simulink model "observer"  (R2022b)
settings: Solver=VariableStepAuto  StartTime=0.0  StopTime=5000  RelTol=1e-3
libraries: mssSimulink x2
settings Model: Creator=ADMIN  LastModifiedBy=ADMIN

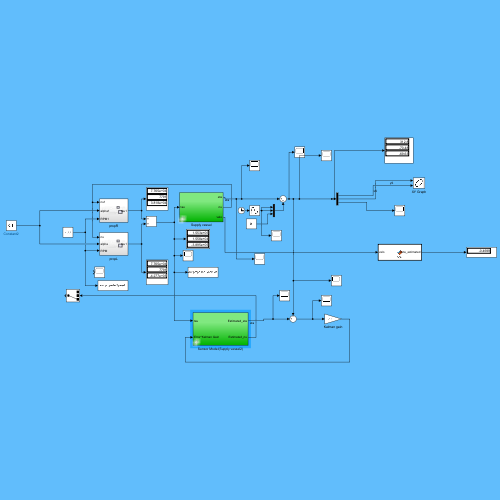
[thumbnail: Simulink's stored preview of the top-level diagram]
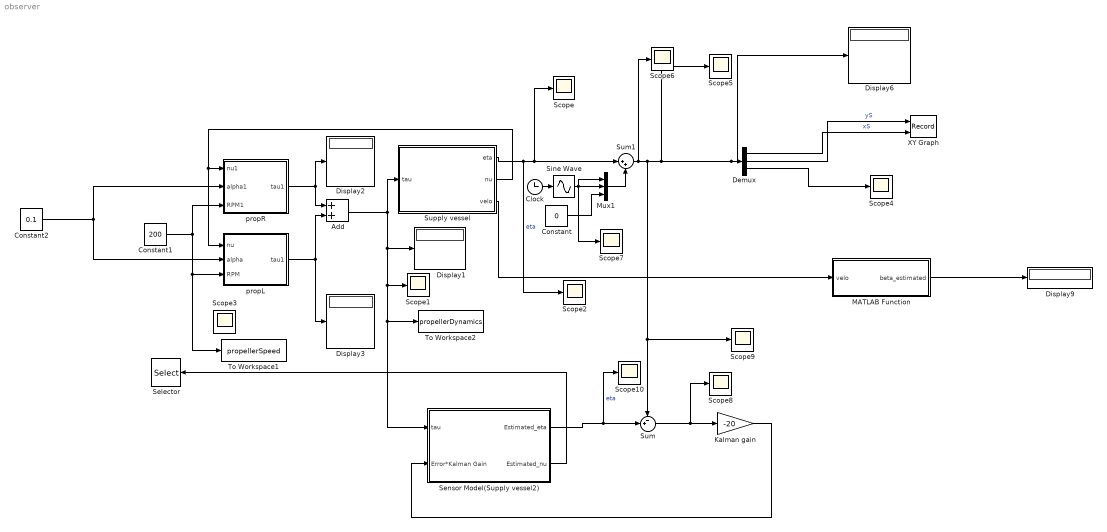
== system observer ==
  Add : Sum
  Clock : Clock
  Constant : Constant  Value=0
  Constant1 : Constant  Value=200
  Constant2 : Constant  Value=0.1
  Demux : Demux  Outputs=3
  Display{1..3,6,9} (5 alike) : Display
  Kalman gain : Gain  Gain=-20
  MATLAB Function : MATLAB Function  TreatAsAtomicUnit=on
  Mux1 : Mux  Inputs=3
  Scope{,1..10} (11 alike) : Scope
  Selector : Selector  InputPortWidth=3  IndexOptions=Index vector (dialog)  Indices=[3]  OutputSizes=1
  Sensor Model(Supply vessel2) : Subsystem  AncestorBlock=mssSimulink/Marine craft models/Supply vessel
      settings: LibrarySourceBlock=mssSimulink/Marine craft models/Supply vessel
  Sine Wave : Sin  TimeSource=Use external signal  SampleTime=0
  Sum : Sum  Inputs=-+|
  Sum1 : Sum  Inputs=|++
  Supply vessel : Subsystem  AncestorBlock=mssSimulink/Marine craft models/Supply vessel
      settings: LibrarySourceBlock=mssSimulink/Marine craft models/Supply vessel
  To Workspace1 : ToWorkspace  VariableName=propellerSpeed  SaveFormat=Timeseries  SampleTime=-1
  To Workspace2 : ToWorkspace  VariableName=propellerDynamics  SaveFormat=Timeseries  SampleTime=-1
  XY Graph : Record  FileSettingsInternal="{\"entries\":[{\"content\":{\"excelSettings\":{\"content\":{},\"type\":\"Streamout.ExcelSettings\"}},\"type\":\"Streamout.FileSettingStorage\",\"uuid\":\"745f10b0-d431-460f-8bac-5fec13218052\"}],\"packageUris\":[\"http://schema.mathworks.com/mf0/streamout_blocks/R2020a\"],\"version\":\"1.0\"}"  Layout=[1 1]  SignalsInternal="{\"entries\":[{\"content\":{\"signals\":[{\"content\":{\"blockPath\":[\"untitled/XY Graph\"],\"channel\":[],\"dimensions\":[1],\"domain\":\"untitled/XY Graph\",\"lineColor\":\"#edb120\",\"plots\":[],\"port\":1,\"sid\":[\"\"],\"signalID\":6053,\"signalName\":\"yS\"},\"type\":\"RecordBlkView.Signal\",\"uuid\":\"76aacf64-0f69-4baf-8ee2-86f53dc3926d\"},{\"content\":{\"blockPath\":[\"untitled/XY Graph\"],\"channel\":[],\"dimensions\":[1],\"domain\":\"untitled/XY Graph\",\"lineColor\":\"#7e2f8e\",\"plots\":[],\"port\":2,\"sid\":[\"\"],\"signalID\":6057,\"signalName\":\"xS\"},\"type\":\"RecordBlkView.Signal\",\"uuid\":\"9f0f96a2-05ba-4d7f-9a6e-25fee0664970\"}]},\"type\":\"RecordBlkView.InputSignals\",\"uuid\":\"3a7a1a35-8a4d-4271-a4b4-a2beea98fdd3\"}],\"packageUris\":[\"http://schema.mathworks.com/mf0/streamout_blocks/R2020a\"],\"version\":\"1.0\"}"  VisualizationBindings="{\"xyplotplugin\":{\"info\":[{\"series\":[],\"subplotID\":1}]}}"  CompatibilityTag=XY
  propL : Subsystem
  propR : Subsystem
  wires:
  Sum1/1 -> Scope6/1, Scope5/1, Demux/1, Display6/1, Sum/1, Scope9/1
  Sine Wave/1 -> Scope7/1, Mux1/2, Mux1/1
  Mux1/1 -> Sum1/2
  propL/1(tau1) -> Add/2, Display3/1
  Sensor Model(Supply vessel2)/2(Estimated_nu) -> Selector/1
  Demux/1 -> XY Graph/2  "xS"
  Sum/1 -> Scope8/1, Kalman gain/1
  Sensor Model(Supply vessel2)/1(Estimated_eta) -> Scope10/1, Sum/2  "eta"
  Supply vessel/1(eta) -> Sum1/1, Scope/1, Scope2/1  "eta"
  Kalman gain/1 -> Sensor Model(Supply vessel2)/2(Error*Kalman Gain)
  Supply vessel/3(velo) -> MATLAB Function/1(velo)
  Demux/3 -> Scope4/1
  Demux/2 -> XY Graph/1  "yS"
  Supply vessel/2(nu) -> propR/1(nu1), propL/1(nu)
  Clock/1 -> Sine Wave/1
  propR/1(tau1) -> Display2/1, Add/1
  Add/1 -> Sensor Model(Supply vessel2)/1(tau), To Workspace2/1, Scope1/1, Display1/1, Supply vessel/1(tau)
  MATLAB Function/1(beta_estimated) -> Display9/1
  Constant/1 -> Mux1/3
  Constant1/1 -> propL/3(RPM), To Workspace1/1, propR/3(RPM1)
  Constant2/1 -> propL/2(alpha), propR/2(alpha1)

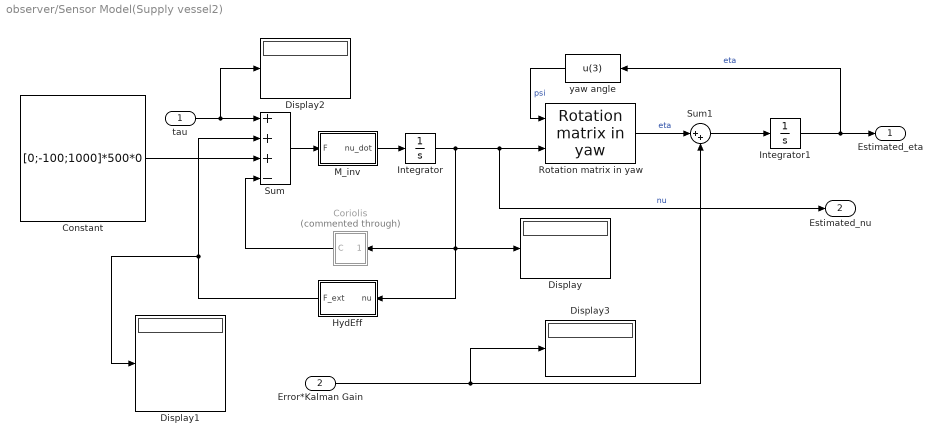
== system observer/Sensor Model(Supply vessel2) ==
  tau : Inport
  Error*Kalman Gain : Inport  Port=2
  Constant : Constant  Value=[0;-100;1000]*500*0
  Coriolis : Subsystem  Commented=through
  Display{,1..3} (4 alike) : Display
  HydEff : Subsystem
  Integrator : Integrator  InitialCondition=[0 1 0]
  Integrator1 : Integrator
  M_inv : Subsystem
  "Rotation matrix in yaw " : mssSimulink/Modelling/Kinematics/Rotation matrix in yaw 
  Sum : Sum  Inputs=+++-  InputSameDT=on  SaturateOnIntegerOverflow=on  OutDataTypeStr=Inherit: Same as first input
  Sum1 : Sum  Inputs=|++
  yaw angle : Fcn  Expr=u(3)
  Estimated_eta : Outport  InitialOutput=0  VectorParamsAs1DForOutWhenUnconnected=off
  Estimated_nu : Outport  Port=2  InitialOutput=0  VectorParamsAs1DForOutWhenUnconnected=off
  wires:
  Sum/1 -> M_inv/1(F)
  M_inv/1(nu_dot) -> Integrator/1
  tau/1 -> Display2/1, Sum/1
  yaw angle/1 -> "Rotation matrix in yaw "/1  "psi"
  Integrator/1 -> Estimated_nu/1, "Rotation matrix in yaw "/2, Display/1, HydEff/1(nu), Coriolis/1(nu)  "nu"
  HydEff/1(F_ext) -> Display1/1, Sum/2
  Coriolis/1(C) -> Sum/4
  Constant/1 -> Sum/3
  Integrator1/1 -> Estimated_eta/1, yaw angle/1  "eta"
  Error*Kalman Gain/1 -> Display3/1, Sum1/2
  Sum1/1 -> Integrator1/1
  "Rotation matrix in yaw "/1 -> Sum1/1  "eta"

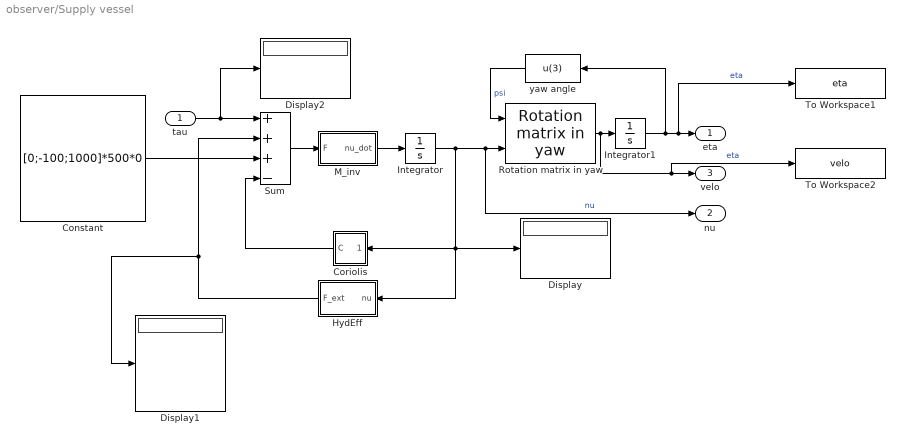
== system observer/Supply vessel ==
  tau : Inport
  Constant : Constant  Value=[0;-100;1000]*500*0
  Coriolis : Subsystem
  Display : Display
  Display1 : Display
  Display2 : Display
  HydEff : Subsystem
  Integrator : Integrator  InitialCondition=[0 1 0]
  Integrator1 : Integrator
  M_inv : Subsystem
  "Rotation matrix in yaw " : mssSimulink/Modelling/Kinematics/Rotation matrix in yaw 
  Sum : Sum  Inputs=+++-  InputSameDT=on  SaturateOnIntegerOverflow=on  OutDataTypeStr=Inherit: Same as first input
  To Workspace1 : ToWorkspace  VariableName=eta  SaveFormat=Timeseries  SampleTime=-1
  To Workspace2 : ToWorkspace  VariableName=velo  SaveFormat=Timeseries  SampleTime=-1
  yaw angle : Fcn  Expr=u(3)
  eta : Outport  InitialOutput=0  VectorParamsAs1DForOutWhenUnconnected=off
  nu : Outport  Port=2  InitialOutput=0  VectorParamsAs1DForOutWhenUnconnected=off
  velo : Outport  Port=3
  wires:
  Sum/1 -> M_inv/1(F)
  M_inv/1(nu_dot) -> Integrator/1
  tau/1 -> Display2/1, Sum/1
  yaw angle/1 -> "Rotation matrix in yaw "/1  "psi"
  Integrator/1 -> Display/1, HydEff/1(nu), Coriolis/1(nu), "Rotation matrix in yaw "/2, nu/1  "nu"
  HydEff/1(F_ext) -> Display1/1, Sum/2
  Coriolis/1(C) -> Sum/4
  Constant/1 -> Sum/3
  Integrator1/1 -> yaw angle/1, To Workspace1/1, eta/1  "eta"
  "Rotation matrix in yaw "/1 -> To Workspace2/1, velo/1, Integrator1/1  "eta"

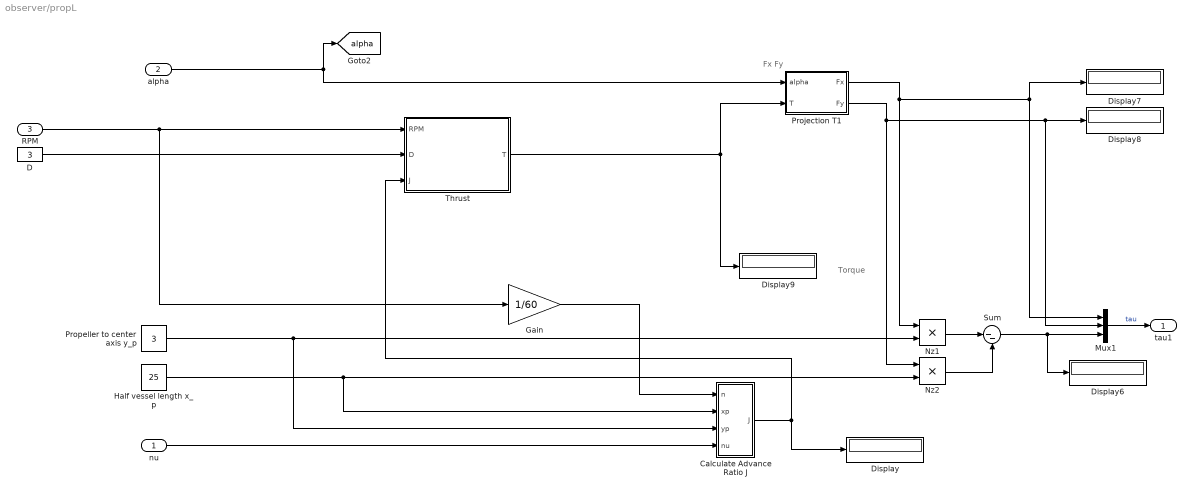
== system observer/propL ==
  note: Fx Fy
  note: Torque
  nu : Inport
  alpha : Inport  Port=2
  RPM : Inport  Port=3
  Calculate Advance Ratio J : Subsystem
  D : Constant  Value=3
  Display{,6..9} (5 alike) : Display
  Gain : Gain  Gain=1/60
  Half vessel length x_p : Constant  Value=25
  Mux1 : Mux  Inputs=3
  Nz1 : Product
  Nz2 : Product
  Projection T1 : MATLAB Function  TreatAsAtomicUnit=on
  Propeller to center axis y_p : Constant  Value=3
  Sum : Sum  Inputs=|--
  Thrust : Subsystem
  tau1 : Outport
  tag scope: alpha=global
  wires:
  Gain/1 -> Calculate Advance Ratio J/1(n)
  Thrust/1(T) -> Projection T1/2(T), Display9/1
  Propeller to center axis y_p/1 -> Calculate Advance Ratio J/3(yp), Nz1/2
  Projection T1/2(Fy) -> Mux1/2, Display8/1, Nz2/1
  RPM/1 -> Gain/1, Thrust/1(RPM)
  Nz2/1 -> Sum/2
  Projection T1/1(Fx) -> Display7/1, Mux1/1, Nz1/1
  Mux1/1 -> tau1/1  "tau"
  alpha/1 -> Projection T1/1(alpha), [alpha]
  D/1 -> Thrust/2(D)
  nu/1 -> Calculate Advance Ratio J/4(nu)
  Half vessel length x_p/1 -> Calculate Advance Ratio J/2(xp), Nz2/2
  Nz1/1 -> Sum/1
  Calculate Advance Ratio J/1(J) -> Thrust/3(J), Display/1
  Sum/1 -> Display6/1, Mux1/3

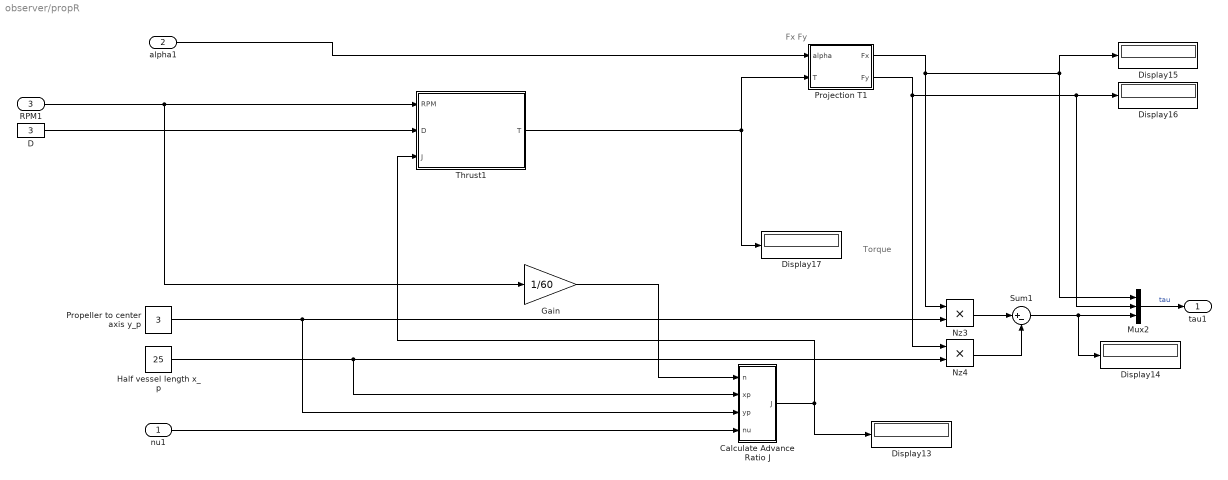
== system observer/propR ==
  note: Fx Fy
  note: Torque
  nu1 : Inport
  alpha1 : Inport  Port=2
  RPM1 : Inport  Port=3
  Calculate Advance Ratio J : Subsystem
  D : Constant  Value=3
  Display{13..17} (5 alike) : Display
  Gain : Gain  Gain=1/60
  Half vessel length x_p : Constant  Value=25
  Mux2 : Mux  Inputs=3
  Nz3 : Product
  Nz4 : Product
  Projection T1 : MATLAB Function  TreatAsAtomicUnit=on
  Propeller to center axis y_p : Constant  Value=3
  Sum1 : Sum  Inputs=|+-
  Thrust1 : Subsystem
  tau1 : Outport
  wires:
  Gain/1 -> Calculate Advance Ratio J/1(n)
  Thrust1/1(T) -> Projection T1/2(T), Display17/1
  Propeller to center axis y_p/1 -> Calculate Advance Ratio J/3(yp), Nz3/2
  Projection T1/2(Fy) -> Mux2/2, Display16/1, Nz4/1
  RPM1/1 -> Gain/1, Thrust1/1(RPM)
  Nz4/1 -> Sum1/2
  Projection T1/1(Fx) -> Display15/1, Mux2/1, Nz3/1
  Mux2/1 -> tau1/1  "tau"
  alpha1/1 -> Projection T1/1(alpha)
  D/1 -> Thrust1/2(D)
  nu1/1 -> Calculate Advance Ratio J/4(nu)
  Half vessel length x_p/1 -> Calculate Advance Ratio J/2(xp), Nz4/2
  Nz3/1 -> Sum1/1
  Calculate Advance Ratio J/1(J) -> Thrust1/3(J), Display13/1
  Sum1/1 -> Display14/1, Mux2/3

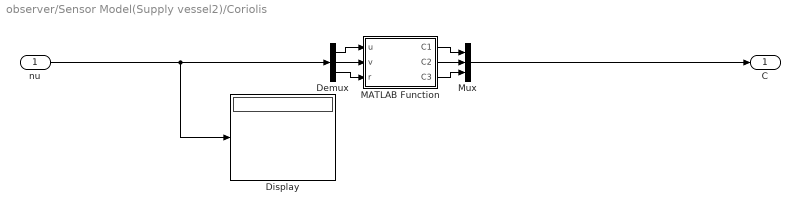
== system observer/Sensor Model(Supply vessel2)/Coriolis ==
  nu : Inport
  Demux : Demux  Outputs=3
  Display : Display
  MATLAB Function : MATLAB Function  TreatAsAtomicUnit=on
  Mux : Mux  Inputs=3
  C : Outport
  wires:
  nu/1 -> Display/1, Demux/1
  MATLAB Function/2(C2) -> Mux/2
  MATLAB Function/3(C3) -> Mux/3
  MATLAB Function/1(C1) -> Mux/1
  Mux/1 -> C/1
  Demux/1 -> MATLAB Function/1(u)
  Demux/2 -> MATLAB Function/2(v)
  Demux/3 -> MATLAB Function/3(r)

== system observer/Sensor Model(Supply vessel2)/HydEff ==
  nu : Inport
  Bus Creator : BusCreator  Inputs=3
  Demux : Demux  Outputs=3
  MATLAB Function : MATLAB Function  TreatAsAtomicUnit=on
  F_ext : Outport
  wires:
  [Mass1] -> MATLAB Function/1(mass)
  MATLAB Function/1(Xh) -> Bus Creator/1
  Bus Creator/1 -> F_ext/1
  MATLAB Function/2(Yh) -> Bus Creator/2
  MATLAB Function/3(Nh) -> Bus Creator/3
  nu/1 -> Demux/1
  Demux/1 -> MATLAB Function/2(u)
  Demux/2 -> MATLAB Function/3(v)
  Demux/3 -> MATLAB Function/4(r)

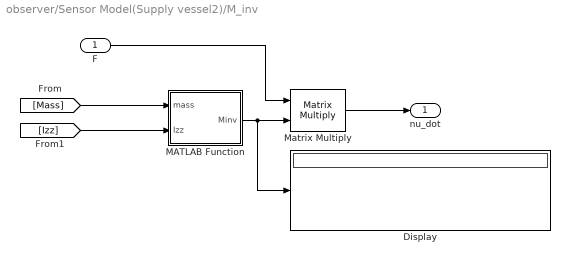
== system observer/Sensor Model(Supply vessel2)/M_inv ==
  F : Inport
  Display : Display
  MATLAB Function : MATLAB Function  TreatAsAtomicUnit=on
  Matrix Multiply : Product  Multiplication=Matrix(*)
  nu_dot : Outport
  wires:
  MATLAB Function/1(Minv) -> Display/1, Matrix Multiply/2
  [Mass] -> MATLAB Function/1(mass)
  [Izz] -> MATLAB Function/2(Izz)
  Matrix Multiply/1 -> nu_dot/1
  F/1 -> Matrix Multiply/1

== system observer/Supply vessel/Coriolis ==
  nu : Inport
  Demux : Demux  Outputs=3
  Display : Display
  MATLAB Function : MATLAB Function  TreatAsAtomicUnit=on
  Mux : Mux  Inputs=3
  C : Outport
  wires:
  nu/1 -> Display/1, Demux/1
  MATLAB Function/2(C2) -> Mux/2
  MATLAB Function/3(C3) -> Mux/3
  MATLAB Function/1(C1) -> Mux/1
  Mux/1 -> C/1
  Demux/1 -> MATLAB Function/1(u)
  Demux/2 -> MATLAB Function/2(v)
  Demux/3 -> MATLAB Function/3(r)

== system observer/Supply vessel/HydEff ==
  nu : Inport
  Bus Creator : BusCreator  Inputs=3
  Demux : Demux  Outputs=3
  MATLAB Function : MATLAB Function  TreatAsAtomicUnit=on
  F_ext : Outport
  wires:
  [Mass] -> MATLAB Function/1(mass)
  MATLAB Function/1(Xh) -> Bus Creator/1
  Bus Creator/1 -> F_ext/1
  MATLAB Function/2(Yh) -> Bus Creator/2
  MATLAB Function/3(Nh) -> Bus Creator/3
  nu/1 -> Demux/1
  Demux/1 -> MATLAB Function/2(u)
  Demux/2 -> MATLAB Function/3(v)
  Demux/3 -> MATLAB Function/4(r)

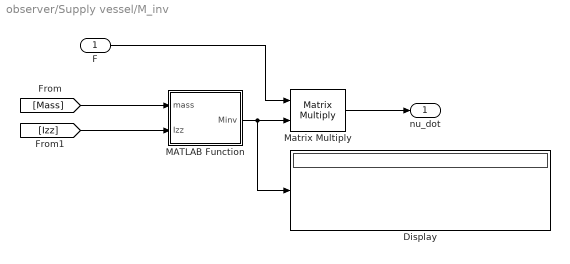
== system observer/Supply vessel/M_inv ==
  F : Inport
  Display : Display
  MATLAB Function : MATLAB Function  TreatAsAtomicUnit=on
  Matrix Multiply : Product  Multiplication=Matrix(*)
  nu_dot : Outport
  wires:
  MATLAB Function/1(Minv) -> Display/1, Matrix Multiply/2
  [Mass] -> MATLAB Function/1(mass)
  [Izz] -> MATLAB Function/2(Izz)
  Matrix Multiply/1 -> nu_dot/1
  F/1 -> Matrix Multiply/1

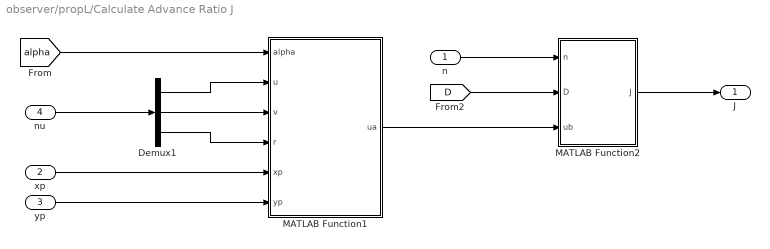
== system observer/propL/Calculate Advance Ratio J ==
  n : Inport
  xp : Inport  Port=2
  yp : Inport  Port=3
  nu : Inport  Port=4
  Demux1 : Demux  Outputs=3
  MATLAB Function1 : MATLAB Function  TreatAsAtomicUnit=on
  MATLAB Function2 : MATLAB Function  TreatAsAtomicUnit=on
  J : Outport
  wires:
  Demux1/3 -> MATLAB Function1/4(r)
  Demux1/2 -> MATLAB Function1/3(v)
  n/1 -> MATLAB Function2/1(n)
  nu/1 -> Demux1/1
  MATLAB Function1/1(ua) -> MATLAB Function2/3(ub)
  Demux1/1 -> MATLAB Function1/2(u)
  [D] -> MATLAB Function2/2(D)
  MATLAB Function2/1(J) -> J/1
  xp/1 -> MATLAB Function1/5(xp)
  yp/1 -> MATLAB Function1/6(yp)
  [alpha] -> MATLAB Function1/1(alpha)

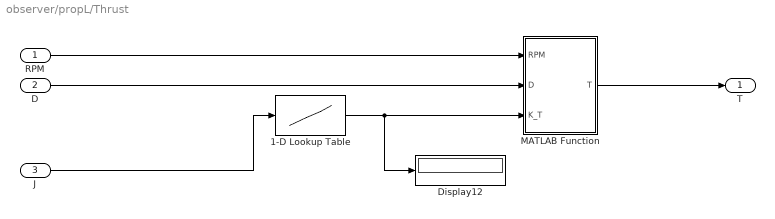
== system observer/propL/Thrust ==
  RPM : Inport
  D : Inport  Port=2
  J : Inport  Port=3
  1-D Lookup Table : Lookup_n-D  NumberOfTableDimensions=1  BreakpointsForDimension1=[0:0.05:1.05]  Table=-0.3*[0:0.05:1.05]+0.35  InternalRulePriority=Speed  RndMeth=Simplest
  Display12 : Display
  MATLAB Function : MATLAB Function  TreatAsAtomicUnit=on
  T : Outport
  wires:
  1-D Lookup Table/1 -> MATLAB Function/3(K_T), Display12/1
  D/1 -> MATLAB Function/2(D)
  MATLAB Function/1(T) -> T/1
  J/1 -> 1-D Lookup Table/1
  RPM/1 -> MATLAB Function/1(RPM)

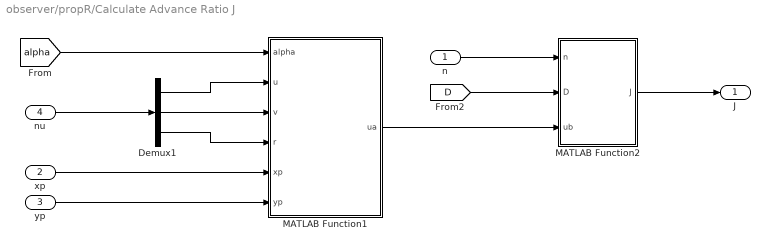
== system observer/propR/Calculate Advance Ratio J ==
  n : Inport
  xp : Inport  Port=2
  yp : Inport  Port=3
  nu : Inport  Port=4
  Demux1 : Demux  Outputs=3
  MATLAB Function1 : MATLAB Function  TreatAsAtomicUnit=on
  MATLAB Function2 : MATLAB Function  TreatAsAtomicUnit=on
  J : Outport
  wires:
  Demux1/3 -> MATLAB Function1/4(r)
  Demux1/2 -> MATLAB Function1/3(v)
  n/1 -> MATLAB Function2/1(n)
  nu/1 -> Demux1/1
  MATLAB Function1/1(ua) -> MATLAB Function2/3(ub)
  Demux1/1 -> MATLAB Function1/2(u)
  [D] -> MATLAB Function2/2(D)
  MATLAB Function2/1(J) -> J/1
  xp/1 -> MATLAB Function1/5(xp)
  yp/1 -> MATLAB Function1/6(yp)
  [alpha] -> MATLAB Function1/1(alpha)

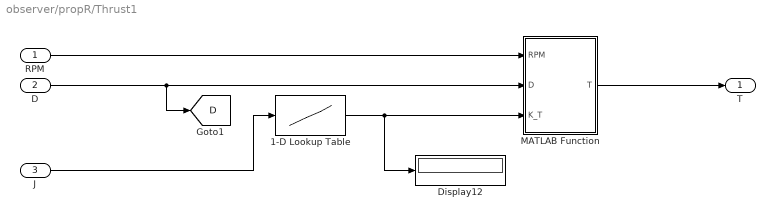
== system observer/propR/Thrust1 ==
  RPM : Inport
  D : Inport  Port=2
  J : Inport  Port=3
  1-D Lookup Table : Lookup_n-D  NumberOfTableDimensions=1  BreakpointsForDimension1=[0:0.05:1.05]  Table=-0.3*[0:0.05:1.05]+0.35  InternalRulePriority=Speed  RndMeth=Simplest
  Display12 : Display
  MATLAB Function : MATLAB Function  TreatAsAtomicUnit=on
  T : Outport
  tag scope: D=global
  wires:
  1-D Lookup Table/1 -> MATLAB Function/3(K_T), Display12/1
  D/1 -> [D], MATLAB Function/2(D)
  MATLAB Function/1(T) -> T/1
  J/1 -> 1-D Lookup Table/1
  RPM/1 -> MATLAB Function/1(RPM)

== matlab function observer/propR/Thrust1/MATLAB Function ==
  data: RPM input; D input; K_T input; T output
function T = fcn(RPM, D, K_T)

RPS = RPM/60;

rho = 1020; % water density

T = K_T*rho*RPS^2*D^4;

== matlab function observer/propR/Projection T1 ==
  data: alpha input; T input; Fx output; Fy output
function [Fx, Fy] = fcn(alpha, T)

Fx = T*cos(alpha);

Fy = T*sin(alpha);

== matlab function observer/Supply vessel/Coriolis/MATLAB Function ==
  data: u input; C1 output; C2 output; C3 output; v input; r input
function [C1,    C2,    C3]    = fcn(u,v,r)

% u = nu(1);
% v = nu(2);
% r = nu(3);

x_g = 0;
m = 357.0*1014;

C = [0                 0  -m*(x_g*r + v); ...
     0                 0             m*u; ...
     m*(x_g*r + v)  -m*u              0];

Co = C*[u;v;r];
C1 = Co(1);
C2 = Co(2);
C3 = Co(3);

end

% Xc =   h.m*(r*v+h.xG*r^2-h.zG*p*r);  
% Yc = - h.m*u*r;
% Kc =   h.m*h.zG*u*r;
% Nc = - h.m*h.xG*u*r;

== matlab function observer/MATLAB Function ==
  data: velo input; beta_estimated output
function beta_estimated = fcn(velo)

beta_estimated = atan2(velo(2), velo(1));

== matlab function observer/Sensor Model(Supply vessel2)/Coriolis/MATLAB Function ==
  data: u input; C1 output; C2 output; C3 output; v input; r input
function [C1,    C2,    C3]    = fcn(u,v,r)

% u = nu(1);
% v = nu(2);
% r = nu(3);

x_g = 0;
m = 357.0*1014;

C = [0                 0  -m*(x_g*r + v); ...
     0                 0             m*u; ...
     m*(x_g*r + v)  -m*u              0];

Co = C*[u;v;r];
C1 = Co(1);
C2 = Co(2);
C3 = Co(3);

end

% Xc =   h.m*(r*v+h.xG*r^2-h.zG*p*r);  
% Yc = - h.m*u*r;
% Kc =   h.m*h.zG*u*r;
% Nc = - h.m*h.xG*u*r;

== matlab function observer/Sensor Model(Supply vessel2)/HydEff/MATLAB Function ==
  data: mass input; Xh output; Yh output; Nh output; u input; v input; r input
function [Xh, Yh, Nh] = fcn(mass, u, v, r)

%%%%%%%%%%%%%%%%%%%%%%%%%%%%%%%%%%%%%%%%%%%%%%%%%%%%%%%%%%%%%%%%%%%%%%%
% The hydrodynamic derivatives are given in dimensional form, and follow
% from the original publication of Blanke and Christensen 1993.
%%%%%%%%%%%%%%%%%%%%%%%%%%%%%%%%%%%%%%%%%%%%%%%%%%%%%%%%%%%%%%%%%%%%%%%
% Data for surge equation 
h.Xudot  	= -17400.0 ;
h.Xuau     	= -1.96e+003 ;
h.Xvr    	=  0.33 * mass ;
   
% Hydrodynamic coefficients in sway equation
uncertain = 0.3;
h.Yvdot = -393000 * uncertain; 
h.Ypdot = -296000 * uncertain; 
h.Yrdot = -1400000 * uncertain; 
h.Yauv  = -11800 * uncertain; 
h.Yur   =  131000 * uncertain; 
h.Yvav  = -3700 * uncertain; 
h.Yrar   =  0 ;
h.Yvar  = -794000 * uncertain; 
h.Yrav  = -182000 * uncertain; 
h.Ybauv =  10800 * uncertain; % Y_{\phi |v u|}
h.Ybaur =  251000 * uncertain; 
h.Ybuu  = -74 * uncertain; 


% Hydrodynamic coefficients in yaw equation
h.Nvdot =  538000 ;
h.Npdot =  0 ;
h.Nrdot = -38.7e6;
h.Nauv  = -92000 ;
h.Naur  = -4710000 ;
h.Nvav  =  0 ;
h.Nrar  = -202000000 ;
h.Nvar  =  0 ;
h.Nrav  = -15600000 ;
h.Nbauv = -214000 ;
h.Nbuar = -4980000 ;
h.Nbuau = -8000 ;
%%%%%%%%%%%%%%%%%%%%%%%%%%%%%%%%%%%%%%%%%%%%%%%%%%%%%%%%%%%%%%%%%%%%%%%%%%%

au = abs(u);
av = abs(v); 
ar = abs(r);
b = 0;

% Hydrodynamic forces without added mass terms (considered in the M matrix)
Xh  = h.Xuau*u*au+h.Xvr*v*r;

Yh = h.Yauv*au*v + h.Yur*u*r + h.Yvav*v*av + h.Yvar*v*ar + h.Yrav*r*av ...
   + h.Ybauv*b*abs(u*v) + h.Ybaur*b*abs(u*r) + h.Ybuu*b*u^2;

Nh = h.Nauv*au*v + h.Naur*au*r + h.Nrar*r*ar + h.Nrav*r*av...
   +h.Nbauv*b*abs(u*b) + h.Nbuar*b*u*ar + h.Nbuau*b*u*au;

end

== matlab function observer/Sensor Model(Supply vessel2)/M_inv/MATLAB Function ==
  data: Minv output; mass input; Izz input
function Minv = fcn(mass, Izz)

h.m   = mass;    % Mass [Kg]
h.Izz = Izz;     % Yaw Inertia
h.xG  = 0;

%%%%%%%%%%%%%%%%%%%%%%%%%%%%%%%%%%%%%%%%%%%%%%%%%%%%%%%%%%%%%%%%%%%%%%%
% The hydrodynamic derivatives are given in dimensional form, and follow
% from the original publication of Blanke and Christensen 1993.
%%%%%%%%%%%%%%%%%%%%%%%%%%%%%%%%%%%%%%%%%%%%%%%%%%%%%%%%%%%%%%%%%%%%%%%
% Data for surge equation 
h.Xudot  	= -17400.0;
% h.Xuau     	= -1.96e+003;
% h.Xvr    	=  0.33 * mass;
   
% Hydrodynamic coefficients in sway equation
h.Yvdot = -393000; 
h.Ypdot = -296000; 
h.Yrdot = -1400000; 
% h.Yauv  = -11800; 
% h.Yur   =  131000; 
% h.Yvav  = -3700; 
% h.Yrar  =  0;
% h.Yvar  = -794000; 
% h.Yrav  = -182000; 
% h.Ybauv =  10800; % Y_{\phi |v u|}
% h.Ybaur =  251000; 
% h.Ybuu  = -74;


% Hydrodynamic coefficients in yaw equation
h.Nvdot =  538000;
h.Npdot =  0;
h.Nrdot = -38.7e6;
% h.Nauv  = -92000;
% h.Naur  = -4710000;
% h.Nvav  =  0;
% h.Nrar  = -202000000;
% h.Nvar  =  0;
% h.Nrav  = -15600000;
% h.Nbauv = -214000;
% h.Nbuar = -4980000;
% h.Nbuau = -8000;
%%%%%%%%%%%%%%%%%%%%%%%%%%%%%%%%%%%%%%%%%%%%%%%%%%%%%%%%%%%%%%%%%%%%%%%%%%%


M = [(h.m-h.Xudot)                  0                  0; ...
                 0      (h.m-h.Yvdot) (h.m*h.xG-h.Yrdot); ...
                 0 (h.m*h.xG-h.Nvdot)    (h.Izz-h.Nrdot)];

Minv = inv(M);
end

== matlab function observer/propL/Calculate Advance Ratio J/MATLAB Function1 ==
  data: alpha input; u input; v input; ua output; r input; xp input; yp input
function ua = fcn(alpha, u, v ,r , xp , yp)
    
    uax = u + yp*r;     % Uax is velocity of propeller projected on x
    uay = v - xp*r;     % Uay is velocity of propeller projected on y
    phi = atan(uay/uax);    % Angle between ship velocity and x axis
    beta = phi - alpha;     % Angle difference between ship velocity and propeller's thrust

    ua = abs(hypot(uax,uay)*cos(beta)); % project ua on direction velocity of ship
end

== matlab function observer/Supply vessel/M_inv/MATLAB Function ==
  data: Minv output; mass input; Izz input
function Minv = fcn(mass, Izz)

h.m   = mass;    % Mass [Kg]
h.Izz = Izz;     % Yaw Inertia
h.xG  = 0;

%%%%%%%%%%%%%%%%%%%%%%%%%%%%%%%%%%%%%%%%%%%%%%%%%%%%%%%%%%%%%%%%%%%%%%%
% The hydrodynamic derivatives are given in dimensional form, and follow
% from the original publication of Blanke and Christensen 1993.
%%%%%%%%%%%%%%%%%%%%%%%%%%%%%%%%%%%%%%%%%%%%%%%%%%%%%%%%%%%%%%%%%%%%%%%
% Data for surge equation 
h.Xudot  	= -17400.0;
% h.Xuau     	= -1.96e+003;
% h.Xvr    	=  0.33 * mass;
   
% Hydrodynamic coefficients in sway equation
h.Yvdot = -393000; 
h.Ypdot = -296000; 
h.Yrdot = -1400000; 
% h.Yauv  = -11800; 
% h.Yur   =  131000; 
% h.Yvav  = -3700; 
% h.Yrar  =  0;
% h.Yvar  = -794000; 
% h.Yrav  = -182000; 
% h.Ybauv =  10800; % Y_{\phi |v u|}
% h.Ybaur =  251000; 
% h.Ybuu  = -74;


% Hydrodynamic coefficients in yaw equation
h.Nvdot =  538000;
h.Npdot =  0;
h.Nrdot = -38.7e6;
% h.Nauv  = -92000;
% h.Naur  = -4710000;
% h.Nvav  =  0;
% h.Nrar  = -202000000;
% h.Nvar  =  0;
% h.Nrav  = -15600000;
% h.Nbauv = -214000;
% h.Nbuar = -4980000;
% h.Nbuau = -8000;
%%%%%%%%%%%%%%%%%%%%%%%%%%%%%%%%%%%%%%%%%%%%%%%%%%%%%%%%%%%%%%%%%%%%%%%%%%%


M = [(h.m-h.Xudot)                  0                  0; ...
                 0      (h.m-h.Yvdot) (h.m*h.xG-h.Yrdot); ...
                 0 (h.m*h.xG-h.Nvdot)    (h.Izz-h.Nrdot)];

Minv = inv(M);
end

== matlab function observer/Supply vessel/HydEff/MATLAB Function ==
  data: mass input; Xh output; Yh output; Nh output; u input; v input; r input
function [Xh, Yh, Nh] = fcn(mass, u, v, r)

%%%%%%%%%%%%%%%%%%%%%%%%%%%%%%%%%%%%%%%%%%%%%%%%%%%%%%%%%%%%%%%%%%%%%%%
% The hydrodynamic derivatives are given in dimensional form, and follow
% from the original publication of Blanke and Christensen 1993.
%%%%%%%%%%%%%%%%%%%%%%%%%%%%%%%%%%%%%%%%%%%%%%%%%%%%%%%%%%%%%%%%%%%%%%%
% Data for surge equation 
h.Xudot  	= -17400.0 ;
h.Xuau     	= -1.96e+003 ;
h.Xvr    	=  0.33 * mass ;
   
% Hydrodynamic coefficients in sway equation
h.Yvdot = -393000 ; 
h.Ypdot = -296000 ; 
h.Yrdot = -1400000 ; 
h.Yauv  = -11800 ; 
h.Yur   =  131000 ; 
h.Yvav  = -3700 ; 
h.Yrar   =  0 ;
h.Yvar  = -794000 ; 
h.Yrav  = -182000 ; 
h.Ybauv =  10800 ; % Y_{\phi |v u|}
h.Ybaur =  251000 ; 
h.Ybuu  = -74 ; 


% Hydrodynamic coefficients in yaw equation
h.Nvdot =  538000 ;
h.Npdot =  0 ;
h.Nrdot = -38.7e6;
h.Nauv  = -92000 ;
h.Naur  = -4710000 ;
h.Nvav  =  0 ;
h.Nrar  = -202000000 ;
h.Nvar  =  0 ;
h.Nrav  = -15600000 ;
h.Nbauv = -214000 ;
h.Nbuar = -4980000 ;
h.Nbuau = -8000 ;
%%%%%%%%%%%%%%%%%%%%%%%%%%%%%%%%%%%%%%%%%%%%%%%%%%%%%%%%%%%%%%%%%%%%%%%%%%%

au = abs(u);
av = abs(v); 
ar = abs(r);
b = 0;

% Hydrodynamic forces without added mass terms (considered in the M matrix)
Xh  = h.Xuau*u*au+h.Xvr*v*r;

Yh = h.Yauv*au*v + h.Yur*u*r + h.Yvav*v*av + h.Yvar*v*ar + h.Yrav*r*av ...
   + h.Ybauv*b*abs(u*v) + h.Ybaur*b*abs(u*r) + h.Ybuu*b*u^2;

Nh = h.Nauv*au*v + h.Naur*au*r + h.Nrar*r*ar + h.Nrav*r*av...
   +h.Nbauv*b*abs(u*b) + h.Nbuar*b*u*ar + h.Nbuau*b*u*au;

end

== matlab function observer/propL/Calculate Advance Ratio J/MATLAB Function2 ==
  data: n input; D input; ub input; J output
function J = fcn(n,D,ub)
    J =ub/(n*D) ;
end

== matlab function observer/propL/Projection T1 ==
  data: alpha input; T input; Fx output; Fy output
function [Fx, Fy] = fcn(alpha, T)

Fx = T*cos(alpha);

Fy = T*sin(alpha);

== matlab function observer/propL/Thrust/MATLAB Function ==
  data: RPM input; D input; K_T input; T output
function T = fcn(RPM, D, K_T)

RPS = RPM/60;

rho = 1020; % water density

T = K_T*rho*RPS^2*D^4;

== matlab function observer/propR/Calculate Advance Ratio J/MATLAB Function1 ==
  data: alpha input; u input; v input; ua output; r input; xp input; yp input
function ua = fcn(alpha, u, v ,r , xp , yp)
    
    uax = u + yp*r;     % Uax is velocity of propeller projected on x
    uay = v - xp*r;     % Uay is velocity of propeller projected on y
    phi = atan(uay/uax);    % Angle between ship velocity and x axis
    beta = phi - alpha;     % Angle difference between ship velocity and propeller's thrust

    ua = abs(hypot(uax,uay)*cos(beta)); % project ua on direction velocity of ship
end

== matlab function observer/propR/Calculate Advance Ratio J/MATLAB Function2 ==
  data: n input; D input; ub input; J output
function J = fcn(n,D,ub)
    J =ub/(n*D) ;
end
